simulink model "VehCtrl20260630_18B"  (R2018b)
settings: Solver=FixedStepAuto  StartTime=0.0  StopTime=inf  FixedStep=0.005  RelTol=1e-3
InitFcn:
  | mbd_mpc_consistency_checks(bdroot(gcs));
undefined symbols (not defined in the file): ANG_DEAD, BMS_NormalPwr, BrakeDeadZone, BrkPrsByBrkPct_TB_X, BrkPrsByBrkPct_TB_Y, DELAY_DISCHARGE, DELAY_RCUOFF, DRV_BACKWARD, DRV_BRAKE, DRV_FORWARD, DRV_NEUTRAL, DRV_PARK, DRV_UNPARK, DRV_ZEROTURN, EPB_LOCK, EPB_UNLOCK, ExtraLoadPwr, FanOff, fifo_0_vect, fifo_1_vect, HiFanReq, HV_finished, HV_No_Active, HV_POWER_OFF, HV_POWER_ON, HVDown, HVON, KaTLS_v_DrgUp_X_VehSpd, KeFTM_s_Way1OffDlyTime, KeFTM_TK_Way1CoolLv2OffBatTemp, KeFTM_TK_Way1CoolLv2OffMtrTemp, KeFTM_TK_Way1CoolLv2OnBatTemp, KeFTM_TK_Way1CoolLv2OnMtrTemp, KeFTM_TK_Way1CoolLv3OffBatTemp, KeFTM_TK_Way1CoolLv3OffMtrTemp, KeFTM_TK_Way1CoolLv3OnBatTemp, KeFTM_TK_Way1CoolLv3OnMtrTemp, KeFTM_TK_Way1CoolLv4OffBatTemp, KeFTM_TK_Way1CoolLv4OffMtrTemp, KeFTM_TK_Way1CoolLv4OnBatTemp, KeFTM_TK_Way1CoolLv4OnMtrTemp, Kp1, Kp2, LowFanReq, LQFP, MtrCmdGainFL, MtrCmdGainFR, MtrCmdGainRL, MtrCmdGainRR, MtrPwrFactor_RCU, MtrPwrHighToMidThd, MtrPwrLowToMidThd, MtrPwrMidToHighThd, MtrPwrMidToLowThd, MtrTrqMax, PCT_DEAD, Precharge, PTO_1000, PTO_540, pts1_fifo_0_vect ... (+32)
libraries: mbd_mpc574x_ec_toolbox x175, simulink x110, canmsglib x70
(part 4 of 15)

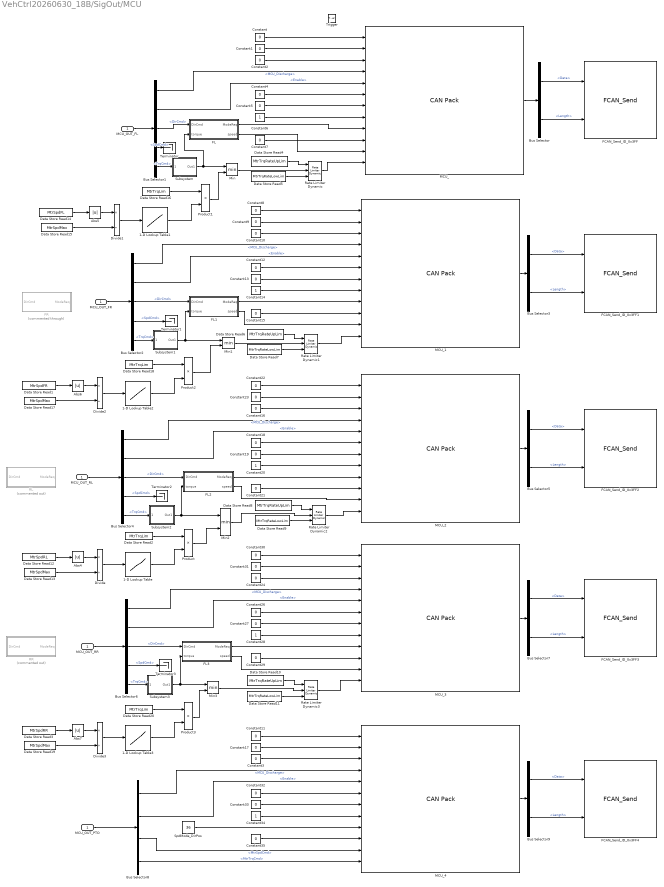
== system VehCtrl20260630_18B/SigOut/MCU ==
  "MCU_OUT_FL " : Inport
  Trigger : TriggerPort  VariantControl=Variant  PortDimensions=1
  1-D Lookup Table{,1..3} (4 alike) : Lookup_n-D  NumberOfTableDimensions=1  BreakpointsForDimension1=[0 0.8 1 10]  Table=[1 1 0 0]  InternalRulePriority=Speed  RndMeth=Simplest  InputSameDT=on
  Abs{4..7} (4 alike) : Abs
  Bus Selector{,3,5,7,9} (5 alike) : BusSelector  OutputSignals=Data,Length
  Bus Selector1 : BusSelector  OutputSignals=MCU_COM.MCU_Discharge,MCU_FL.Enable,MCU_FL.DirCmd,MCU_FL.SpdCmd,MCU_FL.TrqCmd
  Bus Selector2 : BusSelector  OutputSignals=MCU_COM.MCU_Discharge,MCU_FR.Enable,MCU_FR.DirCmd,MCU_FR.SpdCmd,MCU_FR.TrqCmd
  Bus Selector4 : BusSelector  OutputSignals=MCU_COM.MCU_Discharge,MCU_RL.Enable,MCU_RL.DirCmd,MCU_RL.SpdCmd,MCU_RL.TrqCmd
  Bus Selector6 : BusSelector  OutputSignals=MCU_COM.MCU_Discharge,MCU_RR.Enable,MCU_RR.DirCmd,MCU_RR.SpdCmd,MCU_RR.TrqCmd
  Bus Selector8 : BusSelector  OutputSignals=MCU_COM.MCU_Discharge,MCU_PTO.Enable,MCU_PTO.MtrSpdCmd,MCU_PTO.MtrTrqCmd
  Constant{,1..5,7..13,15..19,21..24,26..27,29..33,35} (30 alike) : Constant  Value=0
  Constant{6,14,20,28,34} (5 alike) : Constant
  Data Store Read1 : DataStoreRead  DataStoreName=MtrSpdFR
  Data Store Read{4,6,8,10} (4 alike) : DataStoreRead  DataStoreName=MtrTrqRateUpLim
  Data Store Read{5,7,9,11} (4 alike) : DataStoreRead  DataStoreName=MtrTrqRateLowLim
  Data Store Read12 : DataStoreRead  DataStoreName=MtrSpdRL
  Data Store Read{13,15,17,19} (4 alike) : DataStoreRead  DataStoreName=MtrSpdMax
  Data Store Read14 : DataStoreRead  DataStoreName=MtrSpdFL
  Data Store Read{2,16,18,20} (4 alike) : DataStoreRead  DataStoreName=MtrTrqLim
  Data Store Read3 : DataStoreRead  DataStoreName=MtrSpdRR
  Divide{,1..3} (4 alike) : Product  Inputs=*/
  FCAN_Send_ID_0x3FF : mbd_mpc574x_ec_toolbox/Communication Blocks/CAN Blocks/FCAN_Send  Priority=2  can_instance=2  can_mode=Non-blocking  can_timeout_ms=0  can_mb_idx=60  can_extended_id=on  can_is_remote=off  can_id=C07F3A7  show_adv_opts=off  can_fd_enable=off  can_enable_brs=off  can_fd_padding=0
      settings: SourceProductName=NXP Model-Based Design Toolbox for MPC57xx MCUs
  FCAN_Send_ID_0x3FF1 : mbd_mpc574x_ec_toolbox/Communication Blocks/CAN Blocks/FCAN_Send  Priority=2  can_instance=2  can_mode=Non-blocking  can_timeout_ms=0  can_mb_idx=59  can_extended_id=on  can_is_remote=off  can_id=C07F0A7  show_adv_opts=off  can_fd_enable=off  can_enable_brs=off  can_fd_padding=0
      settings: SourceProductName=NXP Model-Based Design Toolbox for MPC57xx MCUs
  FCAN_Send_ID_0x3FF2 : mbd_mpc574x_ec_toolbox/Communication Blocks/CAN Blocks/FCAN_Send  Priority=2  can_instance=2  can_mode=Non-blocking  can_timeout_ms=0  can_mb_idx=58  can_extended_id=on  can_is_remote=off  can_id=C07F2A7  show_adv_opts=off  can_fd_enable=off  can_enable_brs=off  can_fd_padding=0
      settings: SourceProductName=NXP Model-Based Design Toolbox for MPC57xx MCUs
  FCAN_Send_ID_0x3FF3 : mbd_mpc574x_ec_toolbox/Communication Blocks/CAN Blocks/FCAN_Send  Priority=2  can_instance=2  can_mode=Non-blocking  can_timeout_ms=0  can_mb_idx=57  can_extended_id=on  can_is_remote=off  can_id=C07F1A7  show_adv_opts=off  can_fd_enable=off  can_enable_brs=off  can_fd_padding=0
      settings: SourceProductName=NXP Model-Based Design Toolbox for MPC57xx MCUs
  FCAN_Send_ID_0x3FF4 : mbd_mpc574x_ec_toolbox/Communication Blocks/CAN Blocks/FCAN_Send  Priority=2  can_instance=2  can_mode=Non-blocking  can_timeout_ms=0  can_mb_idx=62  can_extended_id=on  can_is_remote=off  can_id=C07F4A7  show_adv_opts=off  can_fd_enable=off  can_enable_brs=off  can_fd_padding=0
      settings: SourceProductName=NXP Model-Based Design Toolbox for MPC57xx MCUs
  FL : Subsystem
  FL1 : Subsystem
  FL2 : Subsystem
  FL3 : Subsystem
  FR : Subsystem  Commented=through
  MCU_ : canmsglib/CAN Pack  CANdbFile=D:\VCU\VCU_AgriculturalMachinery_ChangChun\CAN协议8.4\MCU\MCU_Sheet1.dbc  MsgList=VCU_MCU_FL  MsgName=VCU_MCU_FL  MsgIDType=Extended (29-bit identifier)  MsgIdentifier=201847719  MsgLength=8  SignalInfo=Reserve$48$12$1$2$1$0$1$0$0$4095$#VCU_BrakePedalSignal$44$1$1$2$1$0$1$0$0$1$#VCU_Canlife$60$4$1$2$1$0$1$0$0$15$#VCU_Discharge$41$1$1$2$1$0$1$0$0$1$#VCU_Enable$40$1$1$2$1$0$1$0$0$1$#VCU_GearSignal$46$2$1$2$1$0$1$0$0$3$#VCU_HandbrakeSignal$45$1$1$2$1$0$1$0$0$1$#VCU_MainContactorStatus$42$1$1$2$1$0$1$0$0$1$#VCU_ModeReq$32$8$1$2$1$0$1$0$0$255$#VCU_PreChargedStatus$43$1$1$2$1$0$1$0$0$1$#VCU_SpdReq$16$16$1$2$1$0$1$-32000$-32000$33535$#VCU_TrqReq$0$16$1$2$1$0$1.000000e-01$-3200$-3200$3.353500e+03$#  NSignals=12  StartBits=str2num('[int32(48);int32(44);int32(60);int32(41);int32(40);int32(46);int32(45);int32(42);int32(32);int32(43);int32(16);int32(0)]')  SignalSizes=str2num('[int32(12);int32(1);int32(4);int32(1);int32(1);int32(2);int32(1);int32(1);int32(8);int32(1);int32(16);int32(16)]')  ByteOrders=str2num('[int32(1);int32(1);int32(1);int32(1);int32(1);int32(1);int32(1);int32(1);int32(1);int32(1);int32(1);int32(1)]')  DataTypes=str2num('[int32(2);int32(2);int32(2);int32(2);int32(2);int32(2);int32(2);int32(2);int32(2);int32(2);int32(2);int32(2)]')  MultiplexTypes=str2num('[int32(1);int32(1);int32(1);int32(1);int32(1);int32(1);int32(1);int32(1);int32(1);int32(1);int32(1);int32(1)]')  MultiplexValues=str2num('[double(0);double(0);double(0);double(0);double(0);double(0);double(0);double(0);double(0);double(0);double(0);double(0)]')  Factors=str2num('[double(1);double(1);double(1);double(1);double(1);double(1);double(1);double(1);double(1);double(1);double(1);double(1.000000e-01)]')  Offsets=str2num('[double(0);double(0);double(0);double(0);double(0);double(0);double(0);double(0);double(0);double(0);double(-32000);double(-3200)]')  Minimums=str2num('[double(0);double(0);double(0);double(0);double(0);double(0);double(0);double(0);double(0);double(0);double(-32000);double(-3200)]')  Maximums=str2num('[double(4095);double(1);double(15);double(1);double(1);double(3);double(1);double(1);double(255);double(1);double(33535);double(3.353500e+03)]')  Remote=off  ApplyMinMax=off  BusOutput=on
      settings: SourceProductName=Simulink Real-Time  SourceProductBaseCode=XP  DataFormat=CANdb specified signals
  MCU_1 : canmsglib/CAN Pack  CANdbFile=D:\VCU\VCU_AgriculturalMachinery_ChangChun\CAN协议8.4\MCU\MCU_Sheet1.dbc  MsgList=VCU_MCU_FR  MsgName=VCU_MCU_FR  MsgIDType=Extended (29-bit identifier)  MsgIdentifier=201846951  MsgLength=8  SignalInfo=Reserve$48$12$1$2$1$0$1$0$0$4095$#VCU_BrakePedalSignal$44$1$1$2$1$0$1$0$0$1$#VCU_Canlife$60$4$1$2$1$0$1$0$0$15$#VCU_Discharge$41$1$1$2$1$0$1$0$0$1$#VCU_Enable$40$1$1$2$1$0$1$0$0$1$#VCU_GearSignal$46$2$1$2$1$0$1$0$0$3$#VCU_HandbrakeSignal$45$1$1$2$1$0$1$0$0$1$#VCU_MainContactorStatus$42$1$1$2$1$0$1$0$0$1$#VCU_ModeReq$32$8$1$2$1$0$1$0$0$255$#VCU_PreChargedStatus$43$1$1$2$1$0$1$0$0$1$#VCU_SpdReq$16$16$1$2$1$0$1$-32000$-32000$33535$#VCU_TrqReq$0$16$1$2$1$0$1.000000e-01$-3200$-3200$3.353500e+03$#  NSignals=12  StartBits=str2num('[int32(48);int32(44);int32(60);int32(41);int32(40);int32(46);int32(45);int32(42);int32(32);int32(43);int32(16);int32(0)]')  SignalSizes=str2num('[int32(12);int32(1);int32(4);int32(1);int32(1);int32(2);int32(1);int32(1);int32(8);int32(1);int32(16);int32(16)]')  ByteOrders=str2num('[int32(1);int32(1);int32(1);int32(1);int32(1);int32(1);int32(1);int32(1);int32(1);int32(1);int32(1);int32(1)]')  DataTypes=str2num('[int32(2);int32(2);int32(2);int32(2);int32(2);int32(2);int32(2);int32(2);int32(2);int32(2);int32(2);int32(2)]')  MultiplexTypes=str2num('[int32(1);int32(1);int32(1);int32(1);int32(1);int32(1);int32(1);int32(1);int32(1);int32(1);int32(1);int32(1)]')  MultiplexValues=str2num('[double(0);double(0);double(0);double(0);double(0);double(0);double(0);double(0);double(0);double(0);double(0);double(0)]')  Factors=str2num('[double(1);double(1);double(1);double(1);double(1);double(1);double(1);double(1);double(1);double(1);double(1);double(1.000000e-01)]')  Offsets=str2num('[double(0);double(0);double(0);double(0);double(0);double(0);double(0);double(0);double(0);double(0);double(-32000);double(-3200)]')  Minimums=str2num('[double(0);double(0);double(0);double(0);double(0);double(0);double(0);double(0);double(0);double(0);double(-32000);double(-3200)]')  Maximums=str2num('[double(4095);double(1);double(15);double(1);double(1);double(3);double(1);double(1);double(255);double(1);double(33535);double(3.353500e+03)]')  Remote=off  ApplyMinMax=off  BusOutput=on
      settings: SourceProductName=Simulink Real-Time  SourceProductBaseCode=XP  DataFormat=CANdb specified signals
  MCU_2 : canmsglib/CAN Pack  CANdbFile=D:\VCU\VCU_AgriculturalMachinery_ChangChun\CAN协议8.4\MCU\MCU_Sheet1.dbc  MsgList=VCU_MCU_RL  MsgName=VCU_MCU_RL  MsgIDType=Extended (29-bit identifier)  MsgIdentifier=201847463  MsgLength=8  SignalInfo=Reserve$48$12$1$2$1$0$1$0$0$4095$#VCU_BrakePedalSignal$44$1$1$2$1$0$1$0$0$1$#VCU_Canlife$60$4$1$2$1$0$1$0$0$15$#VCU_Discharge$41$1$1$2$1$0$1$0$0$1$#VCU_Enable$40$1$1$2$1$0$1$0$0$1$#VCU_GearSignal$46$2$1$2$1$0$1$0$0$3$#VCU_HandbrakeSignal$45$1$1$2$1$0$1$0$0$1$#VCU_MainContactorStatus$42$1$1$2$1$0$1$0$0$1$#VCU_ModeReq$32$8$1$2$1$0$1$0$0$255$#VCU_PreChargedStatus$43$1$1$2$1$0$1$0$0$1$#VCU_SpdReq$16$16$1$2$1$0$1$-32000$-32000$33535$#VCU_TrqReq$0$16$1$2$1$0$1.000000e-01$-3200$-3200$3.353500e+03$#  NSignals=12  StartBits=str2num('[int32(48);int32(44);int32(60);int32(41);int32(40);int32(46);int32(45);int32(42);int32(32);int32(43);int32(16);int32(0)]')  SignalSizes=str2num('[int32(12);int32(1);int32(4);int32(1);int32(1);int32(2);int32(1);int32(1);int32(8);int32(1);int32(16);int32(16)]')  ByteOrders=str2num('[int32(1);int32(1);int32(1);int32(1);int32(1);int32(1);int32(1);int32(1);int32(1);int32(1);int32(1);int32(1)]')  DataTypes=str2num('[int32(2);int32(2);int32(2);int32(2);int32(2);int32(2);int32(2);int32(2);int32(2);int32(2);int32(2);int32(2)]')  MultiplexTypes=str2num('[int32(1);int32(1);int32(1);int32(1);int32(1);int32(1);int32(1);int32(1);int32(1);int32(1);int32(1);int32(1)]')  MultiplexValues=str2num('[double(0);double(0);double(0);double(0);double(0);double(0);double(0);double(0);double(0);double(0);double(0);double(0)]')  Factors=str2num('[double(1);double(1);double(1);double(1);double(1);double(1);double(1);double(1);double(1);double(1);double(1);double(1.000000e-01)]')  Offsets=str2num('[double(0);double(0);double(0);double(0);double(0);double(0);double(0);double(0);double(0);double(0);double(-32000);double(-3200)]')  Minimums=str2num('[double(0);double(0);double(0);double(0);double(0);double(0);double(0);double(0);double(0);double(0);double(-32000);double(-3200)]')  Maximums=str2num('[double(4095);double(1);double(15);double(1);double(1);double(3);double(1);double(1);double(255);double(1);double(33535);double(3.353500e+03)]')  Remote=off  ApplyMinMax=off  BusOutput=on
      settings: SourceProductName=Simulink Real-Time  SourceProductBaseCode=XP  DataFormat=CANdb specified signals
  MCU_3 : canmsglib/CAN Pack  CANdbFile=D:\VCU\VCU_AgriculturalMachinery_ChangChun\CAN协议8.4\MCU\MCU_Sheet1.dbc  MsgList=VCU_MCU_RR  MsgName=VCU_MCU_RR  MsgIDType=Extended (29-bit identifier)  MsgIdentifier=201847207  MsgLength=8  SignalInfo=Reserve$48$12$1$2$1$0$1$0$0$4095$#VCU_BrakePedalSignal$44$1$1$2$1$0$1$0$0$1$#VCU_Canlife$60$4$1$2$1$0$1$0$0$15$#VCU_Discharge$41$1$1$2$1$0$1$0$0$1$#VCU_Enable$40$1$1$2$1$0$1$0$0$1$#VCU_GearSignal$46$2$1$2$1$0$1$0$0$3$#VCU_HandbrakeSignal$45$1$1$2$1$0$1$0$0$1$#VCU_MainContactorStatus$42$1$1$2$1$0$1$0$0$1$#VCU_ModeReq$32$8$1$2$1$0$1$0$0$255$#VCU_PreChargedStatus$43$1$1$2$1$0$1$0$0$1$#VCU_SpdReq$16$16$1$2$1$0$1$-32000$-32000$33535$#VCU_TrqReq$0$16$1$2$1$0$1.000000e-01$-3200$-3200$3.353500e+03$#  NSignals=12  StartBits=str2num('[int32(48);int32(44);int32(60);int32(41);int32(40);int32(46);int32(45);int32(42);int32(32);int32(43);int32(16);int32(0)]')  SignalSizes=str2num('[int32(12);int32(1);int32(4);int32(1);int32(1);int32(2);int32(1);int32(1);int32(8);int32(1);int32(16);int32(16)]')  ByteOrders=str2num('[int32(1);int32(1);int32(1);int32(1);int32(1);int32(1);int32(1);int32(1);int32(1);int32(1);int32(1);int32(1)]')  DataTypes=str2num('[int32(2);int32(2);int32(2);int32(2);int32(2);int32(2);int32(2);int32(2);int32(2);int32(2);int32(2);int32(2)]')  MultiplexTypes=str2num('[int32(1);int32(1);int32(1);int32(1);int32(1);int32(1);int32(1);int32(1);int32(1);int32(1);int32(1);int32(1)]')  MultiplexValues=str2num('[double(0);double(0);double(0);double(0);double(0);double(0);double(0);double(0);double(0);double(0);double(0);double(0)]')  Factors=str2num('[double(1);double(1);double(1);double(1);double(1);double(1);double(1);double(1);double(1);double(1);double(1);double(1.000000e-01)]')  Offsets=str2num('[double(0);double(0);double(0);double(0);double(0);double(0);double(0);double(0);double(0);double(0);double(-32000);double(-3200)]')  Minimums=str2num('[double(0);double(0);double(0);double(0);double(0);double(0);double(0);double(0);double(0);double(0);double(-32000);double(-3200)]')  Maximums=str2num('[double(4095);double(1);double(15);double(1);double(1);double(3);double(1);double(1);double(255);double(1);double(33535);double(3.353500e+03)]')  Remote=off  ApplyMinMax=off  BusOutput=on
      settings: SourceProductName=Simulink Real-Time  SourceProductBaseCode=XP  DataFormat=CANdb specified signals
  MCU_4 : canmsglib/CAN Pack  CANdbFile=D:\VCU\VCU_AgriculturalMachinery_ChangChun\CAN协议8.4\MCU\MCU_Sheet1.dbc  MsgList=VCU_MCU_PTO  MsgName=VCU_MCU_PTO  MsgIDType=Extended (29-bit identifier)  MsgIdentifier=201847975  MsgLength=8  SignalInfo=Reserve$48$12$1$2$1$0$1$0$0$4095$#VCU_BrakePedalSignal$44$1$1$2$1$0$1$0$0$1$#VCU_Canlife$60$4$1$2$1$0$1$0$0$15$#VCU_Discharge$41$1$1$2$1$0$1$0$0$1$#VCU_Enable$40$1$1$2$1$0$1$0$0$1$#VCU_GearSignal$46$2$1$2$1$0$1$0$0$3$#VCU_HandbrakeSignal$45$1$1$2$1$0$1$0$0$1$#VCU_MainContactorStatus$42$1$1$2$1$0$1$0$0$1$#VCU_ModeReq$32$8$1$2$1$0$1$0$0$255$#VCU_PreChargedStatus$43$1$1$2$1$0$1$0$0$1$#VCU_SpdReq$16$16$1$2$1$0$1$-32000$-32000$33535$#VCU_TrqReq$0$16$1$2$1$0$1.000000e-01$-3200$-3200$3.353500e+03$#  NSignals=12  StartBits=str2num('[int32(48);int32(44);int32(60);int32(41);int32(40);int32(46);int32(45);int32(42);int32(32);int32(43);int32(16);int32(0)]')  SignalSizes=str2num('[int32(12);int32(1);int32(4);int32(1);int32(1);int32(2);int32(1);int32(1);int32(8);int32(1);int32(16);int32(16)]')  ByteOrders=str2num('[int32(1);int32(1);int32(1);int32(1);int32(1);int32(1);int32(1);int32(1);int32(1);int32(1);int32(1);int32(1)]')  DataTypes=str2num('[int32(2);int32(2);int32(2);int32(2);int32(2);int32(2);int32(2);int32(2);int32(2);int32(2);int32(2);int32(2)]')  MultiplexTypes=str2num('[int32(1);int32(1);int32(1);int32(1);int32(1);int32(1);int32(1);int32(1);int32(1);int32(1);int32(1);int32(1)]')  MultiplexValues=str2num('[double(0);double(0);double(0);double(0);double(0);double(0);double(0);double(0);double(0);double(0);double(0);double(0)]')  Factors=str2num('[double(1);double(1);double(1);double(1);double(1);double(1);double(1);double(1);double(1);double(1);double(1);double(1.000000e-01)]')  Offsets=str2num('[double(0);double(0);double(0);double(0);double(0);double(0);double(0);double(0);double(0);double(0);double(-32000);double(-3200)]')  Minimums=str2num('[double(0);double(0);double(0);double(0);double(0);double(0);double(0);double(0);double(0);double(0);double(-32000);double(-3200)]')  Maximums=str2num('[double(4095);double(1);double(15);double(1);double(1);double(3);double(1);double(1);double(255);double(1);double(33535);double(3.353500e+03)]')  Remote=off  ApplyMinMax=off  BusOutput=on
      settings: SourceProductName=Simulink Real-Time  SourceProductBaseCode=XP  DataFormat=CANdb specified signals
  MCU_OUT_FR : InportShadow
  MCU_OUT_PTO : InportShadow
  MCU_OUT_RL : InportShadow
  MCU_OUT_RR : InportShadow
  Min{,1..3} (4 alike) : MinMax  Inputs=2
  Product{,1..3} (4 alike) : Product
  RL : Subsystem  Commented=on
  RR : Subsystem  Commented=on
  Rate Limiter Dynamic{,1..3} (4 alike) : simulink/Discontinuities/Rate Limiter Dynamic
      settings: SourceProductName=Simulink
  SpdMode_DirPos : Constant  Value=36  OutDataTypeStr=uint8
  Subsystem : Subsystem
  Subsystem1 : Subsystem
  Subsystem2 : Subsystem
  Subsystem3 : Subsystem
  Terminator{,1..3} (4 alike) : Terminator
  wires:
  MCU_/1 -> Bus Selector/1
  "MCU_OUT_FL "/1 -> Bus Selector1/1
  Bus Selector/1 -> FCAN_Send_ID_0x3FF/1  "<Data>"
  Bus Selector/2 -> FCAN_Send_ID_0x3FF/2  "<Length>"
  Bus Selector1/2 -> MCU_/5  "<Enable>"
  Constant/1 -> MCU_/1
  MCU_OUT_FR/1 -> Bus Selector2/1
  Constant1/1 -> MCU_/2
  Constant2/1 -> MCU_/3
  Bus Selector1/1 -> MCU_/4  "<MCU_Discharge>"
  Constant4/1 -> MCU_/6
  Constant5/1 -> MCU_/7
  Constant6/1 -> MCU_/8
  Constant7/1 -> MCU_/10
  Constant15/1 -> MCU_1/10
  Constant14/1 -> MCU_1/8
  Constant13/1 -> MCU_1/7
  Constant12/1 -> MCU_1/6
  Bus Selector2/1 -> MCU_1/4  "<MCU_Discharge>"
  Constant10/1 -> MCU_1/3
  Constant9/1 -> MCU_1/2
  Constant8/1 -> MCU_1/1
  Bus Selector2/2 -> MCU_1/5  "<Enable>"
  Bus Selector3/2 -> FCAN_Send_ID_0x3FF1/2  "<Length>"
  Bus Selector3/1 -> FCAN_Send_ID_0x3FF1/1  "<Data>"
  MCU_1/1 -> Bus Selector3/1
  MCU_2/1 -> Bus Selector5/1
  Bus Selector5/1 -> FCAN_Send_ID_0x3FF2/1  "<Data>"
  Bus Selector5/2 -> FCAN_Send_ID_0x3FF2/2  "<Length>"
  Bus Selector4/3 -> FL2/1(DirCmd)  "<DirCmd>"
  Bus Selector4/2 -> MCU_2/5  "<Enable>"
  Constant22/1 -> MCU_2/1
  Constant23/1 -> MCU_2/2
  Constant16/1 -> MCU_2/3
  Bus Selector4/1 -> MCU_2/4  "<MCU_Discharge>"
  Constant18/1 -> MCU_2/6
  Constant19/1 -> MCU_2/7
  Constant20/1 -> MCU_2/8
  Constant21/1 -> MCU_2/10
  MCU_OUT_RL/1 -> Bus Selector4/1
  MCU_OUT_RR/1 -> Bus Selector6/1
  Constant29/1 -> MCU_3/10
  Constant28/1 -> MCU_3/8
  Constant27/1 -> MCU_3/7
  Constant26/1 -> MCU_3/6
  Bus Selector6/1 -> MCU_3/4  "<MCU_Discharge>"
  Constant24/1 -> MCU_3/3
  Constant31/1 -> MCU_3/2
  Constant30/1 -> MCU_3/1
  Bus Selector6/2 -> MCU_3/5  "<Enable>"
  Bus Selector6/3 -> FL3/1(DirCmd)  "<DirCmd>"
  Bus Selector7/2 -> FCAN_Send_ID_0x3FF3/2  "<Length>"
  Bus Selector7/1 -> FCAN_Send_ID_0x3FF3/1  "<Data>"
  MCU_3/1 -> Bus Selector7/1
  MCU_4/1 -> Bus Selector9/1
  Bus Selector9/1 -> FCAN_Send_ID_0x3FF4/1  "<Data>"
  Bus Selector9/2 -> FCAN_Send_ID_0x3FF4/2  "<Length>"
  Bus Selector8/2 -> MCU_4/5  "<Enable>"
  Constant32/1 -> MCU_4/6
  Constant33/1 -> MCU_4/7
  Constant34/1 -> MCU_4/8
  Constant35/1 -> MCU_4/10
  MCU_OUT_PTO/1 -> Bus Selector8/1
  Bus Selector8/1 -> MCU_4/4  "<MCU_Discharge>"
  Constant11/1 -> MCU_4/1
  Constant17/1 -> MCU_4/2
  Constant3/1 -> MCU_4/3
  Bus Selector1/3 -> FL/1(DirCmd)  "<DirCmd>"
  FL/1(ModeReq) -> MCU_/9
  Bus Selector2/3 -> FL1/1(DirCmd)  "<DirCmd>"
  FL1/1(ModeReq) -> MCU_1/9
  FL2/1(ModeReq) -> MCU_2/9
  FL3/1(ModeReq) -> MCU_3/9
  Bus Selector8/4 -> MCU_4/12  "<MtrTrqCmd>"
  SpdMode_DirPos/1 -> MCU_4/9
  Min/1 -> Rate Limiter Dynamic/2
  Bus Selector2/5 -> Subsystem1/1(<TrqCmd>)  "<TrqCmd>"
  Rate Limiter Dynamic1/1 -> MCU_1/12
  Bus Selector4/5 -> Subsystem2/1(<TrqCmd>)  "<TrqCmd>"
  Bus Selector8/3 -> MCU_4/11  "<MtrSpdCmd>"
  Rate Limiter Dynamic/1 -> MCU_/12
  Data Store Read4/1 -> Rate Limiter Dynamic/1
  Data Store Read5/1 -> Rate Limiter Dynamic/3
  Min1/1 -> Rate Limiter Dynamic1/2
  Data Store Read7/1 -> Rate Limiter Dynamic1/3
  Data Store Read6/1 -> Rate Limiter Dynamic1/1
  Min2/1 -> Rate Limiter Dynamic2/2
  Data Store Read9/1 -> Rate Limiter Dynamic2/3
  Data Store Read8/1 -> Rate Limiter Dynamic2/1
  Rate Limiter Dynamic2/1 -> MCU_2/12
  Min3/1 -> Rate Limiter Dynamic3/2
  Data Store Read11/1 -> Rate Limiter Dynamic3/3
  Data Store Read10/1 -> Rate Limiter Dynamic3/1
  Rate Limiter Dynamic3/1 -> MCU_3/12
  Bus Selector6/5 -> Subsystem3/1(<TrqCmd>)  "<TrqCmd>"
  Product/1 -> Min2/2
  Data Store Read2/1 -> Product/1
  Data Store Read12/1 -> Abs4/1
  Abs4/1 -> Divide/1
  Data Store Read13/1 -> Divide/2
  Divide/1 -> 1-D Lookup Table/1
  1-D Lookup Table/1 -> Product/2
  Divide1/1 -> 1-D Lookup Table1/1
  1-D Lookup Table1/1 -> Product1/2
  Data Store Read16/1 -> Product1/1
  Data Store Read14/1 -> Abs5/1
  Data Store Read15/1 -> Divide1/2
  Abs5/1 -> Divide1/1
  Product1/1 -> Min/2
  Divide2/1 -> 1-D Lookup Table2/1
  1-D Lookup Table2/1 -> Product2/2
  Data Store Read18/1 -> Product2/1
  Data Store Read1/1 -> Abs6/1
  Data Store Read17/1 -> Divide2/2
  Abs6/1 -> Divide2/1
  Product2/1 -> Min1/2
  Divide3/1 -> 1-D Lookup Table3/1
  1-D Lookup Table3/1 -> Product3/2
  Data Store Read20/1 -> Product3/1
  Data Store Read3/1 -> Abs7/1
  Data Store Read19/1 -> Divide3/2
  Abs7/1 -> Divide3/1
  Product3/1 -> Min3/2
  FL/2(speed) -> MCU_/11
  Bus Selector1/4 -> Terminator/1  "<SpdCmd>"
  Bus Selector2/4 -> Terminator1/1  "<SpdCmd>"
  FL1/2(speed) -> MCU_1/11
  FL2/2(speed) -> MCU_2/11
  Bus Selector4/4 -> Terminator2/1  "<SpdCmd>"
  Bus Selector6/4 -> Terminator3/1  "<SpdCmd>"
  FL3/2(speed) -> MCU_3/11
  Subsystem/1(Out1) -> FL/2(torque), Min/1
  Bus Selector1/5 -> Subsystem/1(<TrqCmd>)  "<TrqCmd>"
  Subsystem1/1(Out1) -> FL1/2(torque), Min1/1
  Subsystem2/1(Out1) -> FL2/2(torque), Min2/1
  Subsystem3/1(Out1) -> FL3/2(torque), Min3/1

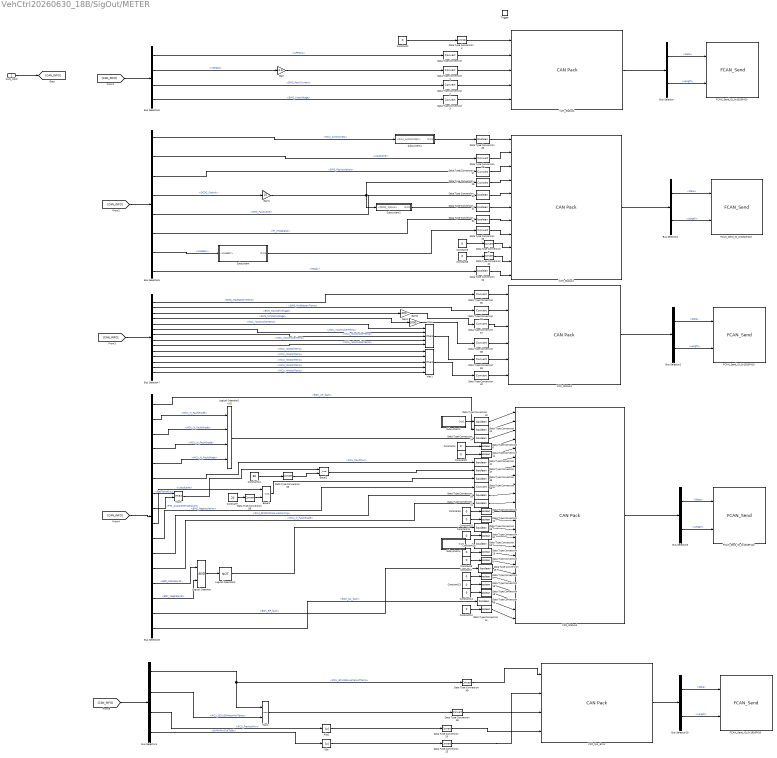
== system VehCtrl20260630_18B/SigOut/METER ==
  "CAN_INFO " : Inport
  Trigger : TriggerPort  VariantControl=Variant  PortDimensions=1
  Abs : Abs
  Abs1 : Abs
  Bus Selector{,1..3,10} (5 alike) : BusSelector  OutputSignals=Data,Length
  Bus Selector4 : BusSelector  OutputSignals=RCU.RCU_MSG_3.RCU_GCUISGInverterActTemp,RCU.RCU_MSG_3.RCU_GCUISGMotorActTemp,RCU.RCU_MSG_2.RCU_RexActPwr,DrMtrPwrOutTotal
  Bus Selector5 : BusSelector  OutputSignals=BMS.DbugBMS_SOC_CaleSOC.APPSOC,VehSpd,BMS.BMS_PackMeasure.BMS_PackCurrent,BMS.BMS_PackMeasure.BMS_LineVoltage
  Bus Selector6 : BusSelector  OutputSignals=RCU.RCU_MSG_1.RCU_ActWorkSts,DAQ.LiqudLevel,BMS.BMS_PackCalc.BMS_PosInsulation,DCDC.DCDC_Optvol,BMS.BMS_PackStateInf.BMS_FaultLevel,BMS.DbugBMS_ESM.IPI_ChrgSignal,CMD.ModeDir,Ready
  Bus Selector7 : BusSelector  OutputSignals=BMS.BMS_ExtremeTemp.BMS_MaxBatteryTemp,BMS.BMS_ExtremeTemp.BMS_MinBatteryTemp,BMS.BMS_ExtremeCellVoltage.BMS_MaxCellVoltage,BMS.BMS_ExtremeCellVoltage.BMS_MinCellVoltage,MCU_FL.MCU2VCU_2.MCU_nControllerTemp,MCU_FR.MCU2VCU_2.MCU_nControllerTemp,MCU_RL.MCU2VCU_2.MCU_nControllerTemp,MCU_RR.MCU2VCU_2.MCU_nControllerTemp,MCU_PTO.MCU2VCU_2.MCU_nControllerTemp,MCU_FL.MCU2VCU_2.MCU_nMotorTemp,MCU_FR.MCU2VCU_2.MCU_nMotorTemp,MCU_RL.MCU2VCU_2.MCU_nMotorTemp,MCU_RR.MCU2VCU_2.MCU_nMotorTemp,MCU_PTO.MCU2VCU_2.MCU_nMotorTemp
  Bus Selector8 : BusSelector  OutputSignals=BDX.AVCU.BDX_AP_fault,MCU_FL.MCU2VCU_3.MCU_N_FaultGrade,MCU_FR.MCU2VCU_3.MCU_N_FaultGrade,MCU_RL.MCU2VCU_3.MCU_N_FaultGrade,MCU_RR.MCU2VCU_3.MCU_N_FaultGrade,RCU.RCU_MSG_1.RCU_RexFltLvl,DAQ.BatTempOut,PTC.signal1.PTC_Coolanttemperature,DAQ.LiqudLevel,BMS.BMS_PackCalc.BMS_NegInsulation,RCU.RCU_MSG_3.RCU_EMSOilPressureWarning,MCU_PTO.MCU2VCU_3.MCU_N_FaultGrade,BMS.DbugBMS_ESM.ESM_PosRelaySt,BMS.DbugBMS_ESM.ESM_NegRelaySt,BDX.AVCU.BDX_BP_fault,BDX.AVCU.BDX_SA_fault
  Constant1 : Constant  Value=20
  Constant{2..14,18} (14 alike) : Constant  Value=0
  Constant24 : Constant  Value=80
  Data Type Conversion{,1..3,5,10,20,23,27..29,33,35..40,43,49,55..56,58} (23 alike) : DataTypeConversion
  Data Type Conversion{6..9,11..16,26,30..32,34,41..42,44..48,50..54,59} (28 alike) : DataTypeConversion  OutDataTypeStr=boolean
  Data Type Conversion4 : DataTypeConversion  OutDataTypeStr=uint16
  Equal1 : RelationalOperator  Operator=<=  OutDataTypeStr=boolean  RndMeth=Simplest
  Equal2 : RelationalOperator  OutDataTypeStr=boolean  RndMeth=Simplest
  FCAN_Send_ID_0x1813F410 : mbd_mpc574x_ec_toolbox/Communication Blocks/CAN Blocks/FCAN_Send  Priority=2  can_instance=2  can_mode=Non-blocking  can_timeout_ms=0  can_mb_idx=3  can_extended_id=on  can_is_remote=off  can_id=1813F410  show_adv_opts=off  can_fd_enable=off  can_enable_brs=off  can_fd_padding=0
      settings: SourceProductName=NXP Model-Based Design Toolbox for MPC57xx MCUs
  FCAN_Send_ID_0x1814F410 : mbd_mpc574x_ec_toolbox/Communication Blocks/CAN Blocks/FCAN_Send  Priority=2  can_instance=2  can_mode=Non-blocking  can_timeout_ms=0  can_mb_idx=7  can_extended_id=on  can_is_remote=off  can_id=1814F410  show_adv_opts=off  can_fd_enable=off  can_enable_brs=off  can_fd_padding=0
      settings: SourceProductName=NXP Model-Based Design Toolbox for MPC57xx MCUs
  FCAN_Send_ID_0x1815F410 : mbd_mpc574x_ec_toolbox/Communication Blocks/CAN Blocks/FCAN_Send  Priority=2  can_instance=2  can_mode=Non-blocking  can_timeout_ms=0  can_mb_idx=11  can_extended_id=on  can_is_remote=off  can_id=1815F410  show_adv_opts=off  can_fd_enable=off  can_enable_brs=off  can_fd_padding=0
      settings: SourceProductName=NXP Model-Based Design Toolbox for MPC57xx MCUs
  FCAN_Send_ID_0x1816F410 : mbd_mpc574x_ec_toolbox/Communication Blocks/CAN Blocks/FCAN_Send  Priority=2  can_instance=2  can_mode=Non-blocking  can_timeout_ms=0  can_mb_idx=15  can_extended_id=on  can_is_remote=off  can_id=1816F410  show_adv_opts=off  can_fd_enable=off  can_enable_brs=off  can_fd_padding=0
      settings: SourceProductName=NXP Model-Based Design Toolbox for MPC57xx MCUs
  FCAN_Send_ID_0x1818F410 : mbd_mpc574x_ec_toolbox/Communication Blocks/CAN Blocks/FCAN_Send  Priority=2  can_instance=2  can_mode=Non-blocking  can_timeout_ms=0  can_mb_idx=19  can_extended_id=on  can_is_remote=off  can_id=1818F410  show_adv_opts=off  can_fd_enable=off  can_enable_brs=off  can_fd_padding=0
      settings: SourceProductName=NXP Model-Based Design Toolbox for MPC57xx MCUs
  Gain : Gain  Gain=3.6
  Gain1 : Gain  Gain=10
  Gain2 : Gain  Gain=1000
  Gain3 : Gain  Gain=1000
  Logical Operator : Logic  AllPortsSameDT=off  OutDataTypeStr=boolean
  Logical Operator1 : Logic  Inputs=4  AllPortsSameDT=off  OutDataTypeStr=boolean
  Logical Operator2 : Logic  Operator=NOT  AllPortsSameDT=off  OutDataTypeStr=boolean
  Max : MinMax  Function=max  Inputs=5
  Max1 : MinMax  Function=max  Inputs=5
  Max2 : MinMax  Function=max  Inputs=2
  Max3 : MinMax  Function=max  Inputs=2
  Subsystem : Subsystem
  Subsystem1 : Subsystem
  Subsystem2 : Subsystem
  Subsystem3 : Subsystem
  Subsystem4 : Subsystem
  V2M_Status1 : canmsglib/CAN Pack  CANdbFile=D:\VCU\VCU_AgriculturalMachinery_ChangChun\VCU_AgriculturalMachinery_260520_ChangChun\CAN协议0520\METER\METER_dbc_backup_sync_20260521_181553.dbc  MsgList=V2M_Status1  MsgName=V2M_Status1  MsgIDType=Extended (29-bit identifier)  MsgIdentifier=403960848  MsgLength=8  SignalInfo=S1_Implement_lifting_height$32$16$1$2$1$0$1$0$0$255$#S1_bms_soc$56$8$1$2$1$0$1$0$0$100$#S1_car_speed$48$8$1$2$1$0$1$0$0$100$#S1_total_current$0$16$1$1$1$0$1$0$-32768$32767$#S1_total_voltage$16$16$1$2$1$0$1$0$0$65535$#  NSignals=5  StartBits=str2num('[int32(32);int32(56);int32(48);int32(0);int32(16)]')  SignalSizes=str2num('[int32(16);int32(8);int32(8);int32(16);int32(16)]')  ByteOrders=str2num('[int32(1);int32(1);int32(1);int32(1);int32(1)]')  DataTypes=str2num('[int32(2);int32(2);int32(2);int32(1);int32(2)]')  MultiplexTypes=str2num('[int32(1);int32(1);int32(1);int32(1);int32(1)]')  MultiplexValues=str2num('[double(0);double(0);double(0);double(0);double(0)]')  Factors=str2num('[double(1);double(1);double(1);double(1);double(1)]')  Offsets=str2num('[double(0);double(0);double(0);double(0);double(0)]')  Minimums=str2num('[double(0);double(0);double(0);double(-32768);double(0)]')  Maximums=str2num('[double(255);double(100);double(100);double(32767);double(65535)]')  Remote=off  ApplyMinMax=off  BusOutput=on
      settings: SourceProductName=Simulink Real-Time  SourceProductBaseCode=XP  DataFormat=CANdb specified signals
  V2M_Status2 : canmsglib/CAN Pack  CANdbFile=D:\VCU\VCU_AgriculturalMachinery_ChangChun\VCU_AgriculturalMachinery_260520_ChangChun\CAN协议0520\METER\METER_dbc.dbc  MsgList=V2M_Status2  MsgName=V2M_Status2  MsgIDType=Extended (29-bit identifier)  MsgIdentifier=404026384  MsgLength=8  SignalInfo=REC_Control_ModeEV_REC$12$1$1$2$1$0$1$0$0$1$#S2_HVO$16$8$1$2$1$0$1$0$0$100$#S2_PosInsulation_R$48$16$1$2$1$0$1$0$0$65535$#S2_battery_Voltage$32$16$1$2$1$0$1.000000e-01$0$0$50$#S2_battery_fault_indicator$1$1$1$2$1$0$1$0$0$1$#S2_battery_voltage_low_icon$13$1$1$2$1$0$1$0$0$1$#S2_charging_gun_indicator$8$1$1$2$1$0$1$0$0$1$#S2_gear$6$2$1$2$1$0$1$0$0$3$#S2_motoCtr_temp_Over$24$1$1$2$1$0$1$0$0$1$#S2_moto_temp_Over$25$1$1$2$1$0$1$0$0$1$#S2_ready_indicator$2$1$1$2$1$0$1$0$0$1$#  NSignals=11  StartBits=str2num('[int32(12);int32(16);int32(48);int32(32);int32(1);int32(13);int32(8);int32(6);int32(24);int32(25);int32(2)]')  SignalSizes=str2num('[int32(1);int32(8);int32(16);int32(16);int32(1);int32(1);int32(1);int32(2);int32(1);int32(1);int32(1)]')  ByteOrders=str2num('[int32(1);int32(1);int32(1);int32(1);int32(1);int32(1);int32(1);int32(1);int32(1);int32(1);int32(1)]')  DataTypes=str2num('[int32(2);int32(2);int32(2);int32(2);int32(2);int32(2);int32(2);int32(2);int32(2);int32(2);int32(2)]')  MultiplexTypes=str2num('[int32(1);int32(1);int32(1);int32(1);int32(1);int32(1);int32(1);int32(1);int32(1);int32(1);int32(1)]')  MultiplexValues=str2num('[double(0);double(0);double(0);double(0);double(0);double(0);double(0);double(0);double(0);double(0);double(0)]')  Factors=str2num('[double(1);double(1);double(1);double(1.000000e-01);double(1);double(1);double(1);double(1);double(1);double(1);double(1)]')  Offsets=str2num('[double(0);double(0);double(0);double(0);double(0);double(0);double(0);double(0);double(0);double(0);double(0)]')  Minimums=str2num('[double(0);double(0);double(0);double(0);double(0);double(0);double(0);double(0);double(0);double(0);double(0)]')  Maximums=str2num('[double(1);double(100);double(65535);double(50);double(1);double(1);double(1);double(3);double(1);double(1);double(1)]')  Remote=off  ApplyMinMax=off  BusOutput=on
      settings: SourceProductName=Simulink Real-Time  SourceProductBaseCode=XP  DataFormat=CANdb specified signals
  V2M_Status3 : canmsglib/CAN Pack  CANdbFile=D:\VCU\VCU_AgriculturalMachinery_ChangChun\VCU_AgriculturalMachinery_260520_ChangChun\CAN协议0520\METER\METER_dbc.dbc  MsgList=V2M_Status3  MsgName=V2M_Status3  MsgIDType=Extended (29-bit identifier)  MsgIdentifier=404091920  MsgLength=8  SignalInfo=S3_bat_temp_max$32$8$1$1$1$0$1$-40$-40$215$#S3_bat_temp_min$40$8$1$1$1$0$1$-40$-40$215$#S3_bat_voltage_max$0$16$1$2$1$0$1$0$0$65535$#S3_bat_voltage_min$16$16$1$2$1$0$1$0$0$65535$#S3_moto_ctr_temp$48$8$1$1$1$0$1$-40$-40$215$#S3_moto_temp$56$8$1$1$1$0$1$-40$-40$215$#  NSignals=6  StartBits=str2num('[int32(32);int32(40);int32(0);int32(16);int32(48);int32(56)]')  SignalSizes=str2num('[int32(8);int32(8);int32(16);int32(16);int32(8);int32(8)]')  ByteOrders=str2num('[int32(1);int32(1);int32(1);int32(1);int32(1);int32(1)]')  DataTypes=str2num('[int32(1);int32(1);int32(2);int32(2);int32(1);int32(1)]')  MultiplexTypes=str2num('[int32(1);int32(1);int32(1);int32(1);int32(1);int32(1)]')  MultiplexValues=str2num('[double(0);double(0);double(0);double(0);double(0);double(0)]')  Factors=str2num('[double(1);double(1);double(1);double(1);double(1);double(1)]')  Offsets=str2num('[double(-40);double(-40);double(0);double(0);double(-40);double(-40)]')  Minimums=str2num('[double(-40);double(-40);double(0);double(0);double(-40);double(-40)]')  Maximums=str2num('[double(215);double(215);double(65535);double(65535);double(215);double(215)]')  Remote=off  ApplyMinMax=off  BusOutput=on
      settings: SourceProductName=Simulink Real-Time  SourceProductBaseCode=XP  DataFormat=CANdb specified signals
  V2M_Status4 : canmsglib/CAN Pack  CANdbFile=D:\VCU\VCU_AgriculturalMachinery_ChangChun\VCU_AgriculturalMachinery_260520_ChangChun\CAN协议0520\METER\METER_dbc.dbc  MsgList=V2M_Status4  MsgName=V2M_Status4  MsgIDType=Extended (29-bit identifier)  MsgIdentifier=404157456  MsgLength=8  SignalInfo=S4_Autonomous_Driving_Status_Indicator_Light_ADN$2$1$1$2$1$0$1$0$0$1$#S4_Chassis_System_Fault_CS$1$1$1$2$1$0$1$0$0$1$#S4_Drive_Fault_Indicator_Light$17$1$1$2$1$0$1$0$0$1$#S4_EC_Fault_Indicator_Light$15$1$1$2$1$0$1$0$0$1$#S4_EWP_Electronic_Water_Pump_Malfunction$21$1$1$2$1$0$1$0$0$1$#S4_Engine_malfunction_indicator_light$31$1$1$2$1$0$1$0$0$1$#S4_High_Water_Temperature_Indicator_Light$19$1$1$2$1$0$1$0$0$1$#S4_Methanol_Low_Fuel_Indicator_Light$27$1$1$2$1$0$1$0$0$1$#S4_NegInsulation_R$48$16$1$2$1$0$1$0$0$65535$#S4_Oil_pressure_warning_light$14$1$1$2$1$0$1$0$0$1$#S4_PT0_Fault_Indicator_Light$13$1$1$2$1$0$1$0$0$1$#S4_PTC1_Fault$20$1$1$2$1$0$1$0$0$1$#S4_PTC2_Fault$3$1$1$2$1$0$1$0$0$1$#S4_Power_Battery_Cut_Off_Indicator_Light$4$1$1$2$1$0$1$0$0$1$#S4_Power_Limit_Indicator_Light$5$1$1$2$1$0$1$0$0$1$#S4_Remote_control_status_indicator_light$30$1$1$2$1$0$1$0$0$1$#S4_Vehicle_System_Fault_Indicator_Light$16$1$1$2$1$0$1$0$0$1$#S4_abs_indicator$18$1$1$2$1$0$1$0$0$1$#S4_brake_sys_fault_alarm$29$1$1$2$1$0$1$0$0$1$#S4_high_beam$10$1$1$2$1$0$1$0$0$1$#S4_left_turn$23$1$1$2$1$0$1$0$0$1$#S4_low_beam$9$1$1$2$1$0$1$0$0$1$#S4_power_steering_fault_lamp$28$1$1$2$1$0$1$0$0$1$#S4_right_turn$22$1$1$2$1$0$1$0$0$1$#  NSignals=24  StartBits=str2num('[int32(2);int32(1);int32(17);int32(15);int32(21);int32(31);int32(19);int32(27);int32(48);int32(14);int32(13);int32(20);int32(3);int32(4);int32(5);int32(30);int32(16);int32(18);int32(29);int32(10);int32(23);int32(9);int32(28);int32(22)]')  SignalSizes=str2num('[int32(1);int32(1);int32(1);int32(1);int32(1);int32(1);int32(1);int32(1);int32(16);int32(1);int32(1);int32(1);int32(1);int32(1);int32(1);int32(1);int32(1);int32(1);int32(1);int32(1);int32(1);int32(1);int32(1);int32(1)]')  ByteOrders=str2num('[int32(1);int32(1);int32(1);int32(1);int32(1);int32(1);int32(1);int32(1);int32(1);int32(1);int32(1);int32(1);int32(1);int32(1);int32(1);int32(1);int32(1);int32(1);int32(1);int32(1);int32(1);int32(1);int32(1);int32(1)]')  DataTypes=str2num('[int32(2);int32(2);int32(2);int32(2);int32(2);int32(2);int32(2);int32(2);int32(2);int32(2);int32(2);int32(2);int32(2);int32(2);int32(2);int32(2);int32(2);int32(2);int32(2);int32(2);int32(2);int32(2);int32(2);int32(2)]')  MultiplexTypes=str2num('[int32(1);int32(1);int32(1);int32(1);int32(1);int32(1);int32(1);int32(1);int32(1);int32(1);int32(1);int32(1);int32(1);int32(1);int32(1);int32(1);int32(1);int32(1);int32(1);int32(1);int32(1);int32(1);int32(1);int32(1)]')  MultiplexValues=str2num('[double(0);double(0);double(0);double(0);double(0);double(0);double(0);double(0);double(0);double(0);double(0);double(0);double(0);double(0);double(0);double(0);double(0);double(0);double(0);double(0);double(0);double(0);double(0);double(0)]')  Factors=str2num('[double(1);double(1);double(1);double(1);double(1);double(1);double(1);double(1);double(1);double(1);double(1);double(1);double(1);double(1);double(1);double(1);double(1);double(1);double(1);double(1);double(1);double(1);double(1);double(1)]')  Offsets=str2num('[double(0);double(0);double(0);double(0);double(0);double(0);double(0);double(0);double(0);double(0);double(0);double(0);double(0);double(0);double(0);double(0);double(0);double(0);double(0);double(0);double(0);double(0);double(0);double(0)]')  Minimums=str2num('[double(0);double(0);double(0);double(0);double(0);double(0);double(0);double(0);double(0);double(0);double(0);double(0);double(0);double(0);double(0);double(0);double(0);double(0);double(0);double(0);double(0);double(0);double(0);double(0)]')  Maximums=str2num('[double(1);double(1);double(1);double(1);double(1);double(1);double(1);double(1);double(65535);double(1);double(1);double(1);double(1);double(1);double(1);double(1);double(1);double(1);double(1);double(1);double(1);double(1);double(1);double(1)]')  Remote=off  ApplyMinMax=off  BusOutput=on
      settings: SourceProductName=Simulink Real-Time  SourceProductBaseCode=XP  DataFormat=CANdb specified signals
  "V2M_Sys_Error " : canmsglib/CAN Pack  CANdbFile=D:\VCU\VCU_AgriculturalMachinery_ChangChun\VCU_AgriculturalMachinery_260520_ChangChun\CAN协议0520\METER\METER_dbc.dbc  MsgList=V2M_Sys_Error  MsgName=V2M_Sys_Error  MsgIDType=Extended (29-bit identifier)  MsgIdentifier=404288528  MsgLength=8  SignalInfo=S6_Generator_Temperature$56$8$1$1$1$0$1$-40$-40$215$#S6_Motor_power$0$8$1$1$1$0$10$0$0$2550$#S6_Range_Extender_Temperature$48$8$1$1$1$0$1$-40$-40$215$#S6_Range_extender_power$8$8$1$1$1$0$10$0$0$2550$#  NSignals=4  StartBits=str2num('[int32(56);int32(0);int32(48);int32(8)]')  SignalSizes=str2num('[int32(8);int32(8);int32(8);int32(8)]')  ByteOrders=str2num('[int32(1);int32(1);int32(1);int32(1)]')  DataTypes=str2num('[int32(1);int32(1);int32(1);int32(1)]')  MultiplexTypes=str2num('[int32(1);int32(1);int32(1);int32(1)]')  MultiplexValues=str2num('[double(0);double(0);double(0);double(0)]')  Factors=str2num('[double(1);double(10);double(1);double(10)]')  Offsets=str2num('[double(-40);double(0);double(-40);double(0)]')  Minimums=str2num('[double(-40);double(0);double(-40);double(0)]')  Maximums=str2num('[double(215);double(2550);double(215);double(2550)]')  Remote=off  ApplyMinMax=off  BusOutput=on
      settings: SourceProductName=Simulink Real-Time  SourceProductBaseCode=XP  DataFormat=CANdb specified signals
  wires:
  "CAN_INFO "/1 -> [CAN_INFO]
  Bus Selector3/2 -> FCAN_Send_ID_0x1816F410/2  "<Length>"
  Bus Selector3/1 -> FCAN_Send_ID_0x1816F410/1  "<Data>"
  V2M_Status4/1 -> Bus Selector3/1
  V2M_Status3/1 -> Bus Selector2/1
  Bus Selector2/1 -> FCAN_Send_ID_0x1815F410/1  "<Data>"
  Bus Selector2/2 -> FCAN_Send_ID_0x1815F410/2  "<Length>"
  Bus Selector1/2 -> FCAN_Send_ID_0x1814F410/2  "<Length>"
  Bus Selector1/1 -> FCAN_Send_ID_0x1814F410/1  "<Data>"
  V2M_Status2/1 -> Bus Selector1/1
  V2M_Status1/1 -> Bus Selector/1
  Bus Selector/1 -> FCAN_Send_ID_0x1813F410/1  "<Data>"
  Bus Selector/2 -> FCAN_Send_ID_0x1813F410/2  "<Length>"
  [CAN_INFO] -> Bus Selector5/1
  [CAN_INFO] -> Bus Selector6/1
  [CAN_INFO] -> Bus Selector7/1
  [CAN_INFO] -> Bus Selector8/1
  Bus Selector5/1 -> Data Type Conversion/1  "<APPSOC>"
  Bus Selector5/2 -> Gain/1  "<VehSpd>"
  Bus Selector5/3 -> Data Type Conversion2/1  "<BMS_PackCurrent>"
  Bus Selector5/4 -> Data Type Conversion3/1  "<BMS_LineVoltage>"
  Data Type Conversion/1 -> V2M_Status1/2
  Data Type Conversion1/1 -> V2M_Status1/3
  Bus Selector6/8 -> Data Type Conversion34/1  "<Ready>"
  Bus Selector6/6 -> Data Type Conversion32/1  "<IPI_ChrgSignal>"
  Bus Selector6/4 -> Gain1/1  "<DCDC_Optvol>"
  Bus Selector6/2 -> Data Type Conversion28/1  "<LiqudLevel>"
  Bus Selector6/3 -> Data Type Conversion27/1  "<BMS_PosInsulation>"
  Bus Selector6/1 -> Subsystem1/1(<RCU_ActWorkSts>)  "<RCU_ActWorkSts>"
  Subsystem1/1(Out1) -> Data Type Conversion26/1
  Subsystem2/1(Out1) -> Data Type Conversion31/1
  Bus Selector7/1 -> Data Type Conversion35/1  "<BMS_MaxBatteryTemp>"
  Bus Selector7/2 -> Data Type Conversion36/1  "<BMS_MinBatteryTemp>"
  Bus Selector7/3 -> Gain2/1  "<BMS_MaxCellVoltage>"
  Bus Selector7/4 -> Gain3/1  "<BMS_MinCellVoltage>"
  Bus Selector7/5 -> Max/1  "<MCU_nControllerTemp>"
  Bus Selector7/6 -> Max/2  "<MCU_nControllerTemp>"
  Bus Selector7/7 -> Max/3  "<MCU_nControllerTemp>"
  Bus Selector7/8 -> Max/4  "<MCU_nControllerTemp>"
  Max/1 -> Data Type Conversion39/1
  Bus Selector7/9 -> Max/5  "<MCU_nControllerTemp>"
  Bus Selector7/10 -> Max1/1  "<MCU_nMotorTemp>"
  Bus Selector7/11 -> Max1/2  "<MCU_nMotorTemp>"
  Bus Selector7/12 -> Max1/3  "<MCU_nMotorTemp>"
  Bus Selector7/13 -> Max1/4  "<MCU_nMotorTemp>"
  Bus Selector7/14 -> Max1/5  "<MCU_nMotorTemp>"
  Max1/1 -> Data Type Conversion40/1
  Bus Selector8/1 -> Data Type Conversion41/1  "<BDX_AP_fault>"
  Subsystem3/1(Out1) -> Data Type Conversion42/1
  Bus Selector8/12 -> Data Type Conversion51/1  "<MCU_N_FaultGrade>"
  Bus Selector8/11 -> Data Type Conversion50/1  "<RCU_EMSOilPressureWarning>"
  Bus Selector8/2 -> Logical Operator1/1  "<MCU_N_FaultGrade>"
  Bus Selector8/3 -> Logical Operator1/2  "<MCU_N_FaultGrade>"
  Bus Selector8/4 -> Logical Operator1/3  "<MCU_N_FaultGrade>"
  Bus Selector8/5 -> Logical Operator1/4  "<MCU_N_FaultGrade>"
  Constant1/1 -> Data Type Conversion58/1
  Bus Selector8/9 -> Equal1/1  "<LiqudLevel>"
  Logical Operator1/1 -> Data Type Conversion54/1
  Bus Selector8/15 -> Data Type Conversion46/1  "<BDX_BP_fault>"
  Bus Selector8/16 -> Data Type Conversion45/1  "<BDX_SA_fault>"
  Subsystem4/1(Out1) -> Data Type Conversion53/1
  Bus Selector8/6 -> Data Type Conversion44/1  "<RCU_RexFltLvl>"
  Bus Selector8/10 -> Data Type Conversion43/1  "<BMS_NegInsulation>"
  Data Type Conversion2/1 -> V2M_Status1/4
  Data Type Conversion3/1 -> V2M_Status1/5
  Bus Selector6/5 -> Data Type Conversion30/1  "<BMS_FaultLevel>"
  Logical Operator2/1 -> Data Type Conversion59/1
  Bus Selector8/7 -> Max3/1  "<BatTempOut>"
  Constant2/1 -> Data Type Conversion4/1
  Data Type Conversion4/1 -> V2M_Status1/1
  Constant3/1 -> Data Type Conversion5/1
  Data Type Conversion5/1 -> V2M_Status2/9
  Constant4/1 -> Data Type Conversion6/1
  Data Type Conversion6/1 -> V2M_Status4/4
  Constant5/1 -> Data Type Conversion7/1
  Data Type Conversion7/1 -> V2M_Status4/12
  Constant6/1 -> Data Type Conversion8/1
  Data Type Conversion8/1 -> V2M_Status4/18
  Constant7/1 -> Data Type Conversion9/1
  Data Type Conversion9/1 -> V2M_Status4/20
  Constant8/1 -> Data Type Conversion10/1
  Data Type Conversion10/1 -> V2M_Status2/10
  Data Type Conversion11/1 -> V2M_Status4/5
  Constant9/1 -> Data Type Conversion11/1
  Data Type Conversion12/1 -> V2M_Status4/13
  Constant10/1 -> Data Type Conversion12/1
  Constant18/1 -> Data Type Conversion13/1
  Constant12/1 -> Data Type Conversion14/1
  Data Type Conversion14/1 -> V2M_Status4/24
  Constant13/1 -> Data Type Conversion15/1
  Constant14/1 -> Data Type Conversion16/1
  Data Type Conversion15/1 -> V2M_Status4/21
  Data Type Conversion16/1 -> V2M_Status4/22
  Data Type Conversion26/1 -> V2M_Status2/1
  Data Type Conversion28/1 -> V2M_Status2/2
  Data Type Conversion27/1 -> V2M_Status2/3
  Data Type Conversion29/1 -> V2M_Status2/4
  Data Type Conversion30/1 -> V2M_Status2/5
  Data Type Conversion31/1 -> V2M_Status2/6
  Data Type Conversion32/1 -> V2M_Status2/7
  Data Type Conversion33/1 -> V2M_Status2/8
  Data Type Conversion34/1 -> V2M_Status2/11
  Data Type Conversion35/1 -> V2M_Status3/1
  Data Type Conversion36/1 -> V2M_Status3/2
  Data Type Conversion37/1 -> V2M_Status3/3
  Data Type Conversion39/1 -> V2M_Status3/5
  Data Type Conversion38/1 -> V2M_Status3/4
  Data Type Conversion40/1 -> V2M_Status3/6
  Data Type Conversion41/1 -> V2M_Status4/2
  Data Type Conversion42/1 -> V2M_Status4/1
  Data Type Conversion43/1 -> V2M_Status4/9
  Data Type Conversion44/1 -> V2M_Status4/6
  Data Type Conversion45/1 -> V2M_Status4/23
  Data Type Conversion46/1 -> V2M_Status4/19
  Data Type Conversion47/1 -> V2M_Status4/7
  Data Type Conversion48/1 -> V2M_Status4/8
  Data Type Conversion50/1 -> V2M_Status4/10
  Equal1/1 -> Data Type Conversion48/1
  Data Type Conversion51/1 -> V2M_Status4/11
  Data Type Conversion52/1 -> V2M_Status4/15
  Data Type Conversion53/1 -> V2M_Status4/16
  Data Type Conversion54/1 -> V2M_Status4/3
  Constant24/1 -> Data Type Conversion56/1
  Data Type Conversion56/1 -> Equal2/2
  Equal2/1 -> Data Type Conversion47/1
  Data Type Conversion58/1 -> Equal1/2
  Bus Selector8/13 -> Logical Operator/1  "<ESM_PosRelaySt>"
  Bus Selector8/14 -> Logical Operator/2  "<ESM_NegRelaySt>"
  Logical Operator/1 -> Logical Operator2/1
  Data Type Conversion59/1 -> V2M_Status4/14
  Gain/1 -> Data Type Conversion1/1
  Data Type Conversion13/1 -> V2M_Status4/17
  Bus Selector8/8 -> Max3/2  "<PTC_Coolanttemperature>"
  Max3/1 -> Equal2/1
  Gain1/1 -> Subsystem2/1(<DCDC_Optvol>), Data Type Conversion29/1
  Constant11/1 -> Data Type Conversion52/1
  Gain2/1 -> Data Type Conversion37/1
  Gain3/1 -> Data Type Conversion38/1
  Bus Selector6/7 -> Subsystem/1(<ModeDir>)  "<ModeDir>"
  Subsystem/1(Out1) -> Data Type Conversion33/1
  Bus Selector4/3 -> Abs1/1  "<RCU_RexActPwr>"
  Data Type Conversion23/1 -> "V2M_Sys_Error "/2
  Data Type Conversion55/1 -> "V2M_Sys_Error "/3
  Data Type Conversion49/1 -> "V2M_Sys_Error "/1
  Data Type Conversion20/1 -> "V2M_Sys_Error "/4
  Bus Selector4/4 -> Abs/1  "<DrMtrPwrOutTotal>"
  Max2/1 -> Data Type Conversion55/1
  Bus Selector4/2 -> Max2/2  "<RCU_GCUISGMotorActTemp>"
  "V2M_Sys_Error "/1 -> Bus Selector10/1
  Bus Selector4/1 -> Data Type Conversion49/1, Max2/1  "<RCU_GCUISGInverterActTemp>"
  [CAN_INFO] -> Bus Selector4/1
  Bus Selector10/1 -> FCAN_Send_ID_0x1818F410/1  "<Data>"
  Bus Selector10/2 -> FCAN_Send_ID_0x1818F410/2  "<Length>"
  Abs/1 -> Data Type Conversion23/1
  Abs1/1 -> Data Type Conversion20/1
